simulink library "SEA_library_observers"  (Simulink 8.3)
settings: Solver=ode45  StartTime=0.0  StopTime=10.0  RelTol=1e-3
values from neighbouring files (symbols this model uses):
  I = this.jointModel.I_m + this.jointModel.I_g    [dataSheetGenerator.m]
undefined symbols (not defined in the file or in its folder): C, Cc, DiscIntNeverNeededParam, K, R
undefined symbols (not defined in the file): My_joint, W2k_output_fixed_rigid_gearbox
libraries: cstblocks x4
settings Model: Creator=joern  LastModifiedBy=joern

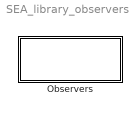
== system SEA_library_observers ==
  Observers : Subsystem

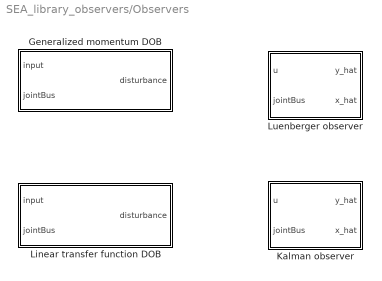
== system SEA_library_observers/Observers ==
  Generalized momentum DOB : Subsystem  mask{jointObj=My_joint, L=60}
      mask prompts: jointObj "Joint Object"; L "Observer gain (disturbance filter frequency in Hz)"
      mask init:
      | % Get linear dynamics matrices
      | [A, B, C, D, I, R, K] = jointObj.getDynamicsMatrices();
      | 
      | % Create a mask matrix to select the proper joint angles and velocities
      | % for a joint model from the joint bus
      | dimSelect = getDimSelectorMatrix(jointObj);
  Kalman observer : Subsystem  mask{jointObj=My_joint, outputIdx=[2], var_u=0.12^2, var_y=1.8e-10}
      mask prompts: jointObj "Joint Object"; outputIdx "Measured outputs (indices)"; var_u "Input noise variance"; var_y "Measurement noise variance"
      mask init:
      | % Get linear dynamics matrices
      | [A, B, C, I, D, K] = jointObj.getDynamicsMatrices();
      | 
      | % Get Kalman observer
      | [kest, L, Cc]	= getKalman(jointObj, outputIdx, var_u, var_y);
      | 
      | % Discretize using Tustin transform
      | kest_tust       = c2d(kest, jointObj.Ts, 'tustin');
      | 
      | % Get demuxing indices
      | demux_N         = size(kest.C,1);               % Kalman state-space block output size
      | demux_yIdx      = 1:length(outputIdx);        	% Estimated outputs indices
      | demux_stateIdx	= length(outputIdx)+1:demux_N;	% Estimated state indices
      | 
      | % Output
      | %disp('Kalman gain L:');
      | %disp(L);
      | %disp('Estimator kest:')
      | %kest
      | %disp('Original dynamic system sys:');
      | %jointObj.getStateSpace()
  Linear transfer function DOB : Subsystem  mask{loadData=off, modelFname=DOB_results.mat, jointObj=W2k_output_fixed_rigid_gearbox, f_c=100, measIdx=7, doPlot=off}
      mask prompts: loadData "Load model/filters/parameters from file"; modelFname "Model/filters file (.mat)"; jointObj "Joint Object"; f_c "Q-filter cut-of frequency [Hz]"; measIdx "Measurement index"; doPlot "Do plot"
      mask init:
      | mask_Linear_Transfer_Function_DOB
      mask Callback loadData:
      | toggleMaskFields(gcbh, 'loadData', 'modelFname', 'on');
      | toggleMaskFields(gcbh, 'loadData', {'jointObj', 'f_c', 'doPlot'}, 'off');
  Luenberger observer : Subsystem  mask{jointObj=My_joint, outputIdx=[2], Q=diag([0 1000 0 0]), R=5e-6, place_gain=4}
      mask prompts: jointObj "Joint Object"; outputIdx "Measured outputs (indices)"; Q "State weighing matrix Q"; R "Input weighing matrix R"; place_gain "Observer place gain"
      mask init:
      | % Get linear dynamics matrices
      | [A, B, C, D] = jointObj.getDynamicsMatrices();
      | 
      | % Get Luenberger observer
      | [sys_hat, L, Cc] = getObserver(jointObj, outputIdx, place_gain, Q, R);
      | 
      | % Discretize using Tustin transform
      | sys_hat_tust = c2d(sys_hat, jointObj.Ts, 'tustin');
      | 
      | % Output
      | %disp('Observer gain L:');
      | %disp(L);
      | %disp('Estimator sys_hat:')
      | %sys_hat
      | %disp('Original dynamic system sys:');
      | %jointObj.getStateSpace()
      | %sys_hat.A - A
      | %sys_hat.B(:,1) - B

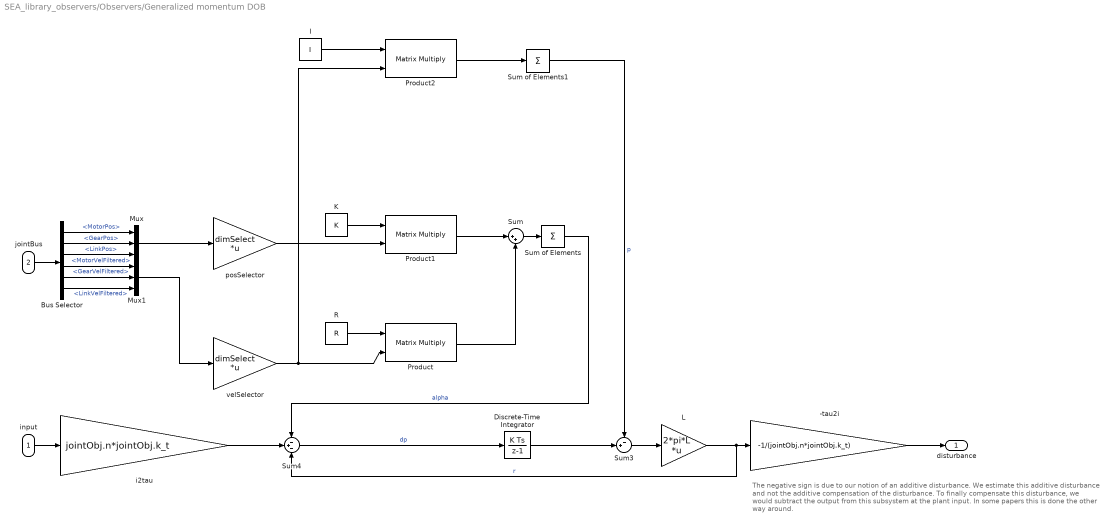
== system SEA_library_observers/Observers/Generalized momentum DOB ==
  note: The negative sign is due to our notion of an additive disturbance.
      | We estimate this additive disturbance and not the additive compensation of the disturbance.
      | To finally compensate this disturbance, we would subtract the output from this subsystem
      | at the plant input.
      | In some papers this is done the other way around.
  input : Inport
  jointBus : Inport  Port=2
  -tau2i : Gain  Gain=-1/(jointObj.n*jointObj.k_t)
  Bus Selector : BusSelector  OutputSignals=MotorPos,GearPos,LinkPos,MotorVelFiltered,GearVelFiltered,LinkVelFiltered
  Discrete-Time Integrator : DiscreteIntegrator  SampleTime=jointObj.Ts  ICPrevOutput=DiscIntNeverNeededParam  ICPrevScaledInput=DiscIntNeverNeededParam
  I : Constant  Value=I
  K : Constant  Value=K
  L : Gain  Gain=2*pi*L  Multiplication=Matrix(K*u)
  Mux : Mux  Inputs=3
  Mux1 : Mux  Inputs=3
  Product : Product  Multiplication=Matrix(*)
  Product1 : Product  Multiplication=Matrix(*)
  Product2 : Product  Multiplication=Matrix(*)
  R : Constant  Value=R
  Sum : Sum  Inputs=|++
  Sum of Elements : Sum  Inputs=+
  Sum of Elements1 : Sum  Inputs=+
  Sum3 : Sum  Inputs=-+|
  Sum4 : Sum  Inputs=-+-
  i2tau : Gain  Gain=jointObj.n*jointObj.k_t
  posSelector : Gain  Gain=dimSelect  Multiplication=Matrix(K*u)
  velSelector : Gain  Gain=dimSelect  Multiplication=Matrix(K*u)
  disturbance : Outport
  wires:
  Sum of Elements1/1 -> Sum3/1  "p"
  Product2/1 -> Sum of Elements1/1
  I/1 -> Product2/1
  Mux/1 -> posSelector/1
  L/1 -> Sum4/3, -tau2i/1  "r"
  Sum of Elements/1 -> Sum4/1  "alpha"
  i2tau/1 -> Sum4/2
  Mux1/1 -> velSelector/1
  Bus Selector/5 -> Mux1/2  "<GearVelFiltered>"
  Bus Selector/4 -> Mux1/1  "<MotorVelFiltered>"
  Bus Selector/6 -> Mux1/3  "<LinkVelFiltered>"
  Bus Selector/1 -> Mux/1  "<MotorPos>"
  Bus Selector/3 -> Mux/3  "<LinkPos>"
  Bus Selector/2 -> Mux/2  "<GearPos>"
  jointBus/1 -> Bus Selector/1
  Sum/1 -> Sum of Elements/1
  posSelector/1 -> Product1/2
  velSelector/1 -> Product/2, Product2/2
  Product/1 -> Sum/2
  Product1/1 -> Sum/1
  K/1 -> Product1/1
  R/1 -> Product/1
  input/1 -> i2tau/1
  Discrete-Time Integrator/1 -> Sum3/2
  Sum3/1 -> L/1
  Sum4/1 -> Discrete-Time Integrator/1  "dp"
  -tau2i/1 -> disturbance/1

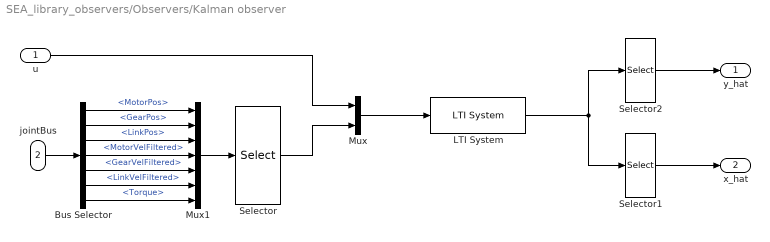
== system SEA_library_observers/Observers/Kalman observer ==
  u : Inport
  jointBus : Inport  Port=2
  Bus Selector : BusSelector  OutputSignals=MotorPos,GearPos,LinkPos,MotorVelFiltered,GearVelFiltered,LinkVelFiltered,Torque
  LTI System : cstblocks/LTI System  sys=kest_tust  IC=[]
  Mux : Mux  Inputs=2
  Mux1 : Mux  Inputs=7
  Selector : Selector  InputPortWidth=size(C,1)  Indices=outputIdx
  Selector1 : Selector  InputPortWidth=demux_N  Indices=demux_stateIdx
  Selector2 : Selector  InputPortWidth=demux_N  Indices=demux_yIdx
  y_hat : Outport
  x_hat : Outport  Port=2
  wires:
  Mux/1 -> LTI System/1
  LTI System/1 -> Selector1/1, Selector2/1
  u/1 -> Mux/1
  Selector1/1 -> x_hat/1
  Selector2/1 -> y_hat/1
  Selector/1 -> Mux/2
  Bus Selector/7 -> Mux1/7  "<Torque>"
  jointBus/1 -> Bus Selector/1
  Bus Selector/4 -> Mux1/4  "<MotorVelFiltered>"
  Bus Selector/2 -> Mux1/2  "<GearPos>"
  Bus Selector/6 -> Mux1/6  "<LinkVelFiltered>"
  Bus Selector/3 -> Mux1/3  "<LinkPos>"
  Bus Selector/5 -> Mux1/5  "<GearVelFiltered>"
  Bus Selector/1 -> Mux1/1  "<MotorPos>"
  Mux1/1 -> Selector/1

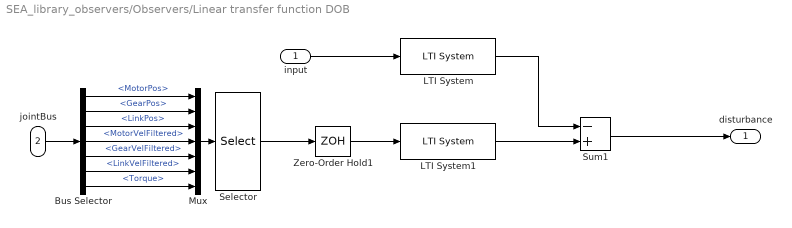
== system SEA_library_observers/Observers/Linear transfer function DOB ==
  input : Inport
  jointBus : Inport  Port=2
  Bus Selector : BusSelector  OutputSignals=MotorPos,GearPos,LinkPos,MotorVelFiltered,GearVelFiltered,LinkVelFiltered,Torque
  LTI System : cstblocks/LTI System  sys=Q_td_tust  IC=[]
  LTI System1 : cstblocks/LTI System  sys=PQ_td_tust  IC=[]
  Mux : Mux  Inputs=7
  Selector : Selector  InputPortWidth=size(C,1)  Indices=measIdx
  Sum1 : Sum  Inputs=-+
  Zero-Order Hold1 : ZeroOrderHold  SampleTime=jointObj.Ts
  disturbance : Outport
  wires:
  Zero-Order Hold1/1 -> LTI System1/1
  Bus Selector/7 -> Mux/7  "<Torque>"
  Selector/1 -> Zero-Order Hold1/1
  LTI System1/1 -> Sum1/2
  LTI System/1 -> Sum1/1
  Sum1/1 -> disturbance/1
  jointBus/1 -> Bus Selector/1
  Bus Selector/4 -> Mux/4  "<MotorVelFiltered>"
  Bus Selector/2 -> Mux/2  "<GearPos>"
  Bus Selector/6 -> Mux/6  "<LinkVelFiltered>"
  Bus Selector/3 -> Mux/3  "<LinkPos>"
  Bus Selector/5 -> Mux/5  "<GearVelFiltered>"
  Bus Selector/1 -> Mux/1  "<MotorPos>"
  Mux/1 -> Selector/1
  input/1 -> LTI System/1

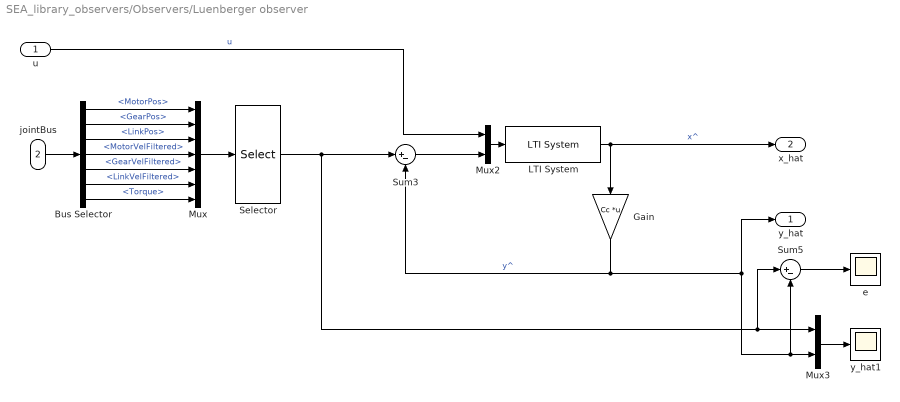
== system SEA_library_observers/Observers/Luenberger observer ==
  u : Inport
  jointBus : Inport  Port=2
  Bus Selector : BusSelector  OutputSignals=MotorPos,GearPos,LinkPos,MotorVelFiltered,GearVelFiltered,LinkVelFiltered,Torque
  Gain : Gain  Gain=Cc  Multiplication=Matrix(K*u)
  LTI System : cstblocks/LTI System  sys=sys_hat_tust  IC=[]
  Mux : Mux  Inputs=7
  Mux2 : Mux  Inputs=2
  Mux3 : Mux  Inputs=2
  Selector : Selector  InputPortWidth=size(C,1)  Indices=outputIdx
  Sum3 : Sum  Inputs=|+-
  Sum5 : Sum  Inputs=|+-
  e : Scope
  y_hat1 : Scope
  y_hat : Outport
  x_hat : Outport  Port=2
  wires:
  Mux3/1 -> y_hat1/1
  Sum5/1 -> e/1
  u/1 -> Mux2/1  "u"
  LTI System/1 -> Gain/1, x_hat/1  "x^"
  Mux2/1 -> LTI System/1
  Selector/1 -> Sum3/1, Mux3/1, Sum5/1
  Sum3/1 -> Mux2/2
  Gain/1 -> y_hat/1, Sum5/2, Mux3/2, Sum3/2  "y^"
  Bus Selector/7 -> Mux/7  "<Torque>"
  jointBus/1 -> Bus Selector/1
  Bus Selector/4 -> Mux/4  "<MotorVelFiltered>"
  Bus Selector/2 -> Mux/2  "<GearPos>"
  Bus Selector/6 -> Mux/6  "<LinkVelFiltered>"
  Bus Selector/3 -> Mux/3  "<LinkPos>"
  Bus Selector/5 -> Mux/5  "<GearVelFiltered>"
  Bus Selector/1 -> Mux/1  "<MotorPos>"
  Mux/1 -> Selector/1
